simulink subsystem "FourTanks_Sub"  (R2023b)
settings: Solver=VariableStepAuto  StartTime=0.0  StopTime=10.0  RelTol=1e-3
values from neighbouring files (symbols this model uses):
  A1 = 28    [init_fourtanks.m]
  A2 = 32    [init_fourtanks.m]
  A3 = 28    [init_fourtanks.m]
  A4 = 32    [init_fourtanks.m]
  g = 981    [init_fourtanks.m]
  k1 = .071    (= 0.071)    [init_fourtanks.m]
  k2 = .057    (= 0.057)    [init_fourtanks.m]
  k3 = .071    (= 0.071)    [init_fourtanks.m]
  k4 = .057    (= 0.057)    [init_fourtanks.m]
  kA = 3.33    [init_fourtanks.m]
  kB = 3.35    [init_fourtanks.m]
undefined symbols (not defined in the file or in its folder): h
settings Model: Creator=HP  LastModifiedBy=HP

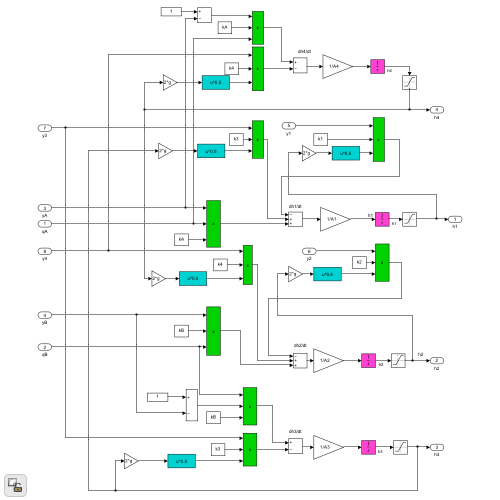
[thumbnail: Simulink's stored preview of the top-level diagram]
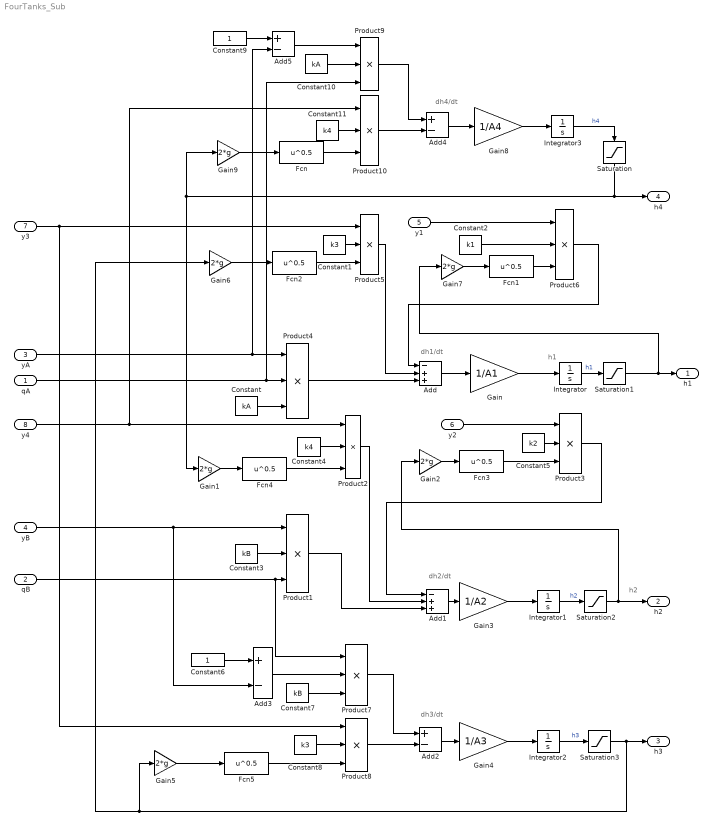
== system FourTanks_Sub ==
  note: h2
  note: h1
  note: dh3/dt
  note: dh4/dt
  note: dh2/dt
  note: dh1/dt
  qA : Inport
  qB : Inport  Port=2
  yA : Inport  Port=3
  yB : Inport  Port=4
  y1 : Inport  Port=5
  y2 : Inport  Port=6
  y3 : Inport  Port=7
  y4 : Inport  Port=8
  Add : Sum  Inputs=-++
  Add1 : Sum  Inputs=-++
  Add{2..5} (4 alike) : Sum  Inputs=+-
  Constant : Constant  Value=kA
  Constant1 : Constant  Value=k3
  Constant10 : Constant  Value=kA
  Constant11 : Constant  Value=k4
  Constant2 : Constant  Value=k1
  Constant3 : Constant  Value=kB
  Constant4 : Constant  Value=k4
  Constant5 : Constant  Value=k2
  Constant6 : Constant
  Constant7 : Constant  Value=kB
  Constant8 : Constant  Value=k3
  Constant9 : Constant
  Fcn{,1..5} (6 alike) : Fcn  Expr=u^0.5
  Gain : Gain  Gain=1/A1
  Gain{1..2,5..7,9} (6 alike) : Gain  Gain=2*g
  Gain3 : Gain  Gain=1/A2
  Gain4 : Gain  Gain=1/A3
  Gain8 : Gain  Gain=1/A4
  Integrator : Integrator  InitialCondition=h(1)
  Integrator1 : Integrator  InitialCondition=h(2)
  Integrator2 : Integrator  InitialCondition=h(3)
  Integrator3 : Integrator  InitialCondition=h(4)
  Product{1..10} (10 alike) : Product  Inputs=3  RndMeth=Zero
  Saturation{,1..3} (4 alike) : Saturate  UpperLimit=inf  LowerLimit=0
  h1 : Outport
  h2 : Outport  Port=2
  h3 : Outport  Port=3
  h4 : Outport  Port=4
  wires:
  Add1/1 -> Gain3/1
  Gain7/1 -> Fcn1/1
  Saturation2/1 -> h2/1, Gain2/1
  Gain8/1 -> Integrator3/1
  y2/1 -> Product3/1
  Constant4/1 -> Product2/2
  Product5/1 -> Add/2
  Constant1/1 -> Product5/2
  Fcn2/1 -> Product5/3
  Add3/1 -> Product7/2
  Constant7/1 -> Product7/3
  Constant3/1 -> Product1/2
  Constant2/1 -> Product6/2
  yB/1 -> Product1/1, Add3/2
  qA/1 -> Product4/2, Product9/3
  qB/1 -> Product1/3, Product7/1
  Constant8/1 -> Product8/2
  Product10/1 -> Add4/2
  Add5/1 -> Product9/1
  Fcn4/1 -> Product2/3
  Gain2/1 -> Fcn3/1
  y4/1 -> Product2/1, Product10/1
  Integrator/1 -> Saturation1/1  "h1"
  Integrator3/1 -> Saturation/1  "h4"
  Constant5/1 -> Product3/2
  Add2/1 -> Gain4/1
  Fcn5/1 -> Product8/3
  y1/1 -> Product6/1
  Gain3/1 -> Integrator1/1
  Gain1/1 -> Fcn4/1
  Gain6/1 -> Fcn2/1
  Integrator2/1 -> Saturation3/1  "h3"
  Constant/1 -> Product4/3
  Add4/1 -> Gain8/1
  Product1/1 -> Add1/3
  Add/1 -> Gain/1
  Gain4/1 -> Integrator2/1
  Constant6/1 -> Add3/1
  Product7/1 -> Add2/1
  Constant11/1 -> Product10/2
  Integrator1/1 -> Saturation2/1  "h2"
  Product8/1 -> Add2/2
  Fcn1/1 -> Product6/3
  yA/1 -> Product4/1, Add5/2
  Product6/1 -> Add/1
  Constant9/1 -> Add5/1
  Product4/1 -> Add/3
  Saturation/1 -> h4/1, Gain9/1, Gain1/1
  Gain5/1 -> Fcn5/1
  Saturation3/1 -> Gain6/1, Gain5/1, h3/1
  Saturation1/1 -> Gain7/1, h1/1
  Gain9/1 -> Fcn/1
  Product2/1 -> Add1/2
  y3/1 -> Product5/1, Product8/1
  Product9/1 -> Add4/1
  Fcn/1 -> Product10/3
  Constant10/1 -> Product9/2
  Gain/1 -> Integrator/1
  Fcn3/1 -> Product3/3
  Product3/1 -> Add1/1
